simulink model "BEML_EMU_TestBench_6Car"  (R2019b)
settings: Solver=VariableStepAuto  StartTime=0.0  StopTime=inf  RelTol=1e-3
PreLoadFcn:
  | set_up_test_modelCB_6Car;
undefined symbols (not defined in the file): Common, IOControls, MaxVehicles, MotionBaseControllerInput, VehicleInputs, VehicleType, Z_CfgVehBus
libraries: TestBenchLib x583, simulink x6
(part 2 of 3)

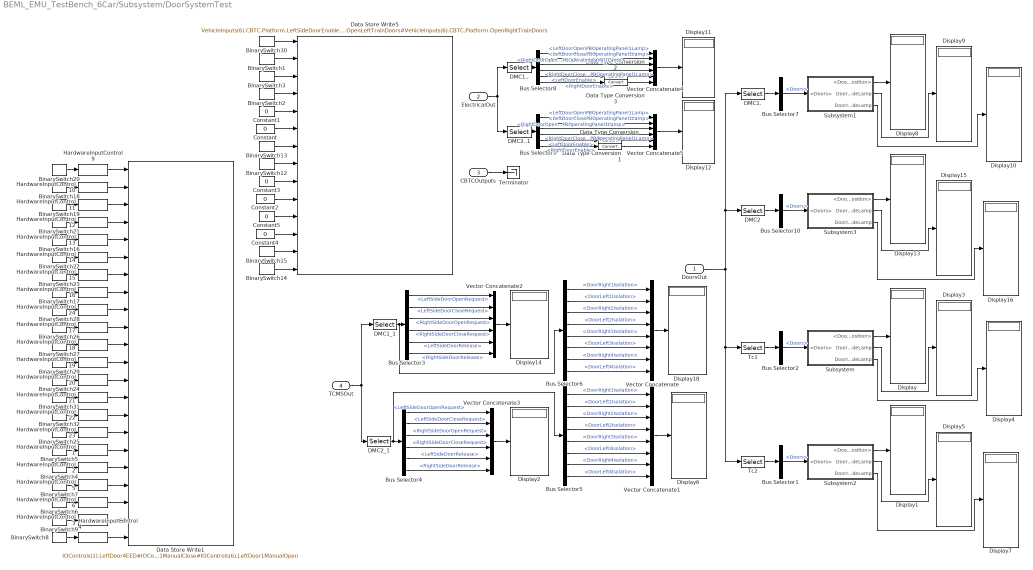
== system BEML_EMU_TestBench_6Car/Subsystem/DoorSystemTest ==
  DoorsOut : Inport
  ElectricalOut : Inport  Port=2
  CBTCOutputs : Inport  Port=3
  TCMSOut : Inport  Port=4
  BinarySwitch{1..9,12..32} (30 alike) : TestBenchLib/BinarySwitch  value=0  init_value=0  block_colour=[0 1 0]  WorkspaceVarName=0
      settings: SourceProductName=Sydac Utilities
  Bus Selector{1..2,7,10} (4 alike) : BusSelector  OutputSignals=Doors
  Bus Selector3 : BusSelector  OutputSignals=Control.DoorSystem.LeftSideDoorOpenRequest,Control.DoorSystem.LeftSideDoorCloseRequest,Control.DoorSystem.RightSideDoorOpenRequest,Control.DoorSystem.RightSideDoorCloseRequest,Control.DoorSystem.LeftSideDoorRelease,Control.DoorSystem.RightSideDoorRelease
  Bus Selector4 : BusSelector  OutputSignals=Control.DoorSystem.LeftSideDoorOpenRequest,Control.DoorSystem.LeftSideDoorCloseRequest,Control.DoorSystem.RightSideDoorOpenRequest,Control.DoorSystem.RightSideDoorCloseRequest,Control.DoorSystem.LeftSideDoorRelease,Control.DoorSystem.RightSideDoorRelease
  Bus Selector5 : BusSelector  OutputSignals=Control.DoorSystem.DoorRight1Isolation,Control.DoorSystem.DoorLeft1Isolation,Control.DoorSystem.DoorRight2Isolation,Control.DoorSystem.DoorLeft2Isolation,Control.DoorSystem.DoorRight3Isolation,Control.DoorSystem.DoorLeft3Isolation,Control.DoorSystem.DoorRight4Isolation,Control.DoorSystem.DoorLeft4Isolation
  Bus Selector6 : BusSelector  OutputSignals=Control.DoorSystem.DoorRight1Isolation,Control.DoorSystem.DoorLeft1Isolation,Control.DoorSystem.DoorRight2Isolation,Control.DoorSystem.DoorLeft2Isolation,Control.DoorSystem.DoorRight3Isolation,Control.DoorSystem.DoorLeft3Isolation,Control.DoorSystem.DoorRight4Isolation,Control.DoorSystem.DoorLeft4Isolation
  Bus Selector8 : BusSelector  OutputSignals=OutputControlStates.LeftDoorOpenPBOperatingPanel1Lamp,OutputControlStates.LeftDoorClosePBOperatingPanel1Lamp,OutputControlStates.RightDoorOpenPBOperatingPanel1Lamp,OutputControlStates.RightDoorClosePBOperatingPanel1Lamp,Doors.LeftDoorEnable,Doors.RightDoorEnable
  Bus Selector9 : BusSelector  OutputSignals=OutputControlStates.LeftDoorOpenPBOperatingPanel1Lamp,OutputControlStates.LeftDoorClosePBOperatingPanel1Lamp,OutputControlStates.RightDoorOpenPBOperatingPanel1Lamp,OutputControlStates.RightDoorClosePBOperatingPanel1Lamp,Doors.LeftDoorEnable,Doors.RightDoorEnable
  Constant{,1..5} (6 alike) : Constant  Value=0
  DMC1. : Selector  InputPortWidth=MaxVehicles  IndexOptions=Index vector (dialog)  Indices=1  OutputSizes=1
  DMC1.. : Selector  InputPortWidth=MaxVehicles  IndexOptions=Index vector (dialog)  Indices=1  OutputSizes=1
  DMC1_1 : Selector  InputPortWidth=MaxVehicles  IndexOptions=Index vector (dialog)  Indices=1  OutputSizes=1
  DMC2 : Selector  InputPortWidth=MaxVehicles  IndexOptions=Index vector (dialog)  Indices=6  OutputSizes=1
  DMC2..1 : Selector  InputPortWidth=MaxVehicles  IndexOptions=Index vector (dialog)  Indices=6  OutputSizes=1
  DMC2_1 : Selector  InputPortWidth=MaxVehicles  IndexOptions=Index vector (dialog)  Indices=6  OutputSizes=1
  Data Store Write1 : DataStoreWrite  Priority=1  DataStoreName=IOControls  DataStoreElements=IOControls(1).LeftDoor4EED#IOControls(1).LeftDoor4ManualClose#IOControls(1).LeftDoor4ManualOpen#IOControls(1).LeftDoor4Lockout#IOControls(1).RightDoor4EED#IOControls(1).RightDoor4ManualClose#IOControls(1).RightDoor4ManualOpen#IOControls(1).RightDoor4Lockout#IOControls(6).LeftDoor4EED#IOControls(6).LeftDoor4ManualClose#IOControls(6).LeftDoor4ManualOpen#IOControls(6).LeftDoor4Lockout#IOControls(6).RightDoor4EED#IOControls(6).RightDoor4ManualClose#IOControls(6).RightDoor4ManualOpen#IOControls(6).RightDoor4Lockout#IOControls(6).RightDoorEAD#IOControls(6).LeftDoorEAD#IOControls(6).RightDoor1ManualClose#IOControls(6).RightDoor1ManualOpen#IOControls(6).LeftDoor1ManualClose#IOControls(6).LeftDoor1ManualOpen
  Data Store Write5 : DataStoreWrite  Priority=1  DataStoreName=VehicleInputs  DataStoreElements=VehicleInputs(6).CBTC.Platform.LeftSideDoorEnable#VehicleInputs(6).CBTC.Platform.RightSideDoorEnable#VehicleInputs(1).CBTC.Platform.LeftSideDoorEnable#VehicleInputs(1).CBTC.Platform.RightSideDoorEnable#VehicleInputs(6).Faults.DoorCloseObstruction#VehicleInputs(6).Faults.DoorOpenObstruction#VehicleInputs(6).CBTC.OnBoard.LeftHoldDoorClose#VehicleInputs(6).CBTC.OnBoard.RightHoldDoorClose#VehicleInputs(1).Faults.DoorCloseObstruction#VehicleInputs(1).Faults.DoorOpenObstruction#VehicleInputs(2).Faults.DoorOpenObstruction#VehicleInputs(2).Faults.DoorCloseObstruction#VehicleInputs(6).CBTC.Platform.OpenLeftTrainDoors#VehicleInputs(6).CBTC.Platform.OpenRightTrainDoors
  Data Type Conversion{,1..3} (4 alike) : DataTypeConversion
  Display{,1..16,18} (18 alike) : Display
  HardwareInputControl{1..6,9..24} (22 alike) : TestBenchLib/HardwareInputControl
      settings: SourceProductName=Sydac Utilities
  Subsystem : Subsystem
  Subsystem1 : Subsystem
  Subsystem2 : Subsystem
  Subsystem3 : Subsystem
  Tc1 : Selector  InputPortWidth=MaxVehicles  IndexOptions=Index vector (dialog)  Indices=2  OutputSizes=1
  Tc2 : Selector  InputPortWidth=MaxVehicles  IndexOptions=Index vector (dialog)  Indices=5  OutputSizes=1
  Terminator : Terminator
  Vector Concatenate : Concatenate  NumInputs=8
  Vector Concatenate1 : Concatenate  NumInputs=8
  Vector Concatenate{2..5} (4 alike) : Concatenate  NumInputs=6
  wires:
  Tc1/1 -> Bus Selector2/1
  BinarySwitch30/1 -> Data Store Write5/1
  Bus Selector2/1 -> Subsystem/1(<Doors>)  "<Doors>"
  Subsystem/1(<DoorPosition>) -> Display/1
  Subsystem2/2(DoorOutsideLamp) -> Display5/1
  Bus Selector1/1 -> Subsystem2/1(<Doors>)  "<Doors>"
  Tc2/1 -> Bus Selector1/1
  DoorsOut/1 -> DMC1./1, DMC2/1, Tc1/1, Tc2/1
  BinarySwitch1/1 -> Data Store Write5/2
  DMC1_1/1 -> Bus Selector6/1, Bus Selector3/1
  TCMSOut/1 -> DMC2_1/1, DMC1_1/1
  Vector Concatenate/1 -> Display18/1
  Vector Concatenate1/1 -> Display6/1
  DMC2_1/1 -> Bus Selector5/1, Bus Selector4/1
  Bus Selector5/1 -> Vector Concatenate1/1  "<DoorRight1Isolation>"
  Bus Selector5/2 -> Vector Concatenate1/2  "<DoorLeft1Isolation>"
  Bus Selector5/3 -> Vector Concatenate1/3  "<DoorRight2Isolation>"
  Bus Selector5/4 -> Vector Concatenate1/4  "<DoorLeft2Isolation>"
  Bus Selector5/5 -> Vector Concatenate1/5  "<DoorRight3Isolation>"
  Bus Selector5/6 -> Vector Concatenate1/6  "<DoorLeft3Isolation>"
  Bus Selector5/7 -> Vector Concatenate1/7  "<DoorRight4Isolation>"
  Bus Selector5/8 -> Vector Concatenate1/8  "<DoorLeft4Isolation>"
  Bus Selector6/1 -> Vector Concatenate/1  "<DoorRight1Isolation>"
  Bus Selector6/2 -> Vector Concatenate/2  "<DoorLeft1Isolation>"
  Bus Selector6/3 -> Vector Concatenate/3  "<DoorRight2Isolation>"
  Bus Selector6/4 -> Vector Concatenate/4  "<DoorLeft2Isolation>"
  Bus Selector6/5 -> Vector Concatenate/5  "<DoorRight3Isolation>"
  Bus Selector6/6 -> Vector Concatenate/6  "<DoorLeft3Isolation>"
  Bus Selector6/7 -> Vector Concatenate/7  "<DoorRight4Isolation>"
  Bus Selector6/8 -> Vector Concatenate/8  "<DoorLeft4Isolation>"
  CBTCOutputs/1 -> Terminator/1
  Bus Selector3/1 -> Vector Concatenate2/1  "<LeftSideDoorOpenRequest>"
  Bus Selector3/2 -> Vector Concatenate2/2  "<LeftSideDoorCloseRequest>"
  Bus Selector3/3 -> Vector Concatenate2/3  "<RightSideDoorOpenRequest>"
  Bus Selector3/4 -> Vector Concatenate2/4  "<RightSideDoorCloseRequest>"
  Bus Selector3/5 -> Vector Concatenate2/5  "<LeftSideDoorRelease>"
  Bus Selector3/6 -> Vector Concatenate2/6  "<RightSideDoorRelease>"
  Vector Concatenate2/1 -> Display14/1
  Vector Concatenate3/1 -> Display2/1
  Bus Selector4/6 -> Vector Concatenate3/6  "<RightSideDoorRelease>"
  Bus Selector4/5 -> Vector Concatenate3/5  "<LeftSideDoorRelease>"
  Bus Selector4/4 -> Vector Concatenate3/4  "<RightSideDoorCloseRequest>"
  Bus Selector4/3 -> Vector Concatenate3/3  "<RightSideDoorOpenRequest>"
  Bus Selector4/2 -> Vector Concatenate3/2  "<LeftSideDoorCloseRequest>"
  Bus Selector4/1 -> Vector Concatenate3/1  "<LeftSideDoorOpenRequest>"
  ElectricalOut/1 -> DMC2..1/1, DMC1../1
  BinarySwitch2/1 -> Data Store Write5/4
  BinarySwitch3/1 -> Data Store Write5/3
  Constant1/1 -> Data Store Write5/5
  Constant/1 -> Data Store Write5/6
  BinarySwitch13/1 -> Data Store Write5/7
  BinarySwitch12/1 -> Data Store Write5/8
  Subsystem/2(DoorOutsideLamp) -> Display3/1
  Subsystem/3(DoorInsideLamp) -> Display4/1
  Subsystem2/1(<DoorPosition>) -> Display1/1
  Subsystem2/3(DoorInsideLamp) -> Display7/1
  Subsystem1/3(DoorInsideLamp) -> Display10/1
  Bus Selector7/1 -> Subsystem1/1(<Doors>)  "<Doors>"
  Subsystem1/2(DoorOutsideLamp) -> Display9/1
  Subsystem1/1(<DoorPosition>) -> Display8/1
  DMC1./1 -> Bus Selector7/1
  DMC1../1 -> Bus Selector8/1
  Bus Selector8/1 -> Vector Concatenate4/1  "<LeftDoorOpenPBOperatingPanel1Lamp>"
  Bus Selector8/2 -> Vector Concatenate4/2  "<LeftDoorClosePBOperatingPanel1Lamp>"
  Vector Concatenate4/1 -> Display11/1
  Bus Selector8/3 -> Vector Concatenate4/3  "<RightDoorOpenPBOperatingPanel1Lamp>"
  Bus Selector8/4 -> Vector Concatenate4/4  "<RightDoorClosePBOperatingPanel1Lamp>"
  Bus Selector9/4 -> Vector Concatenate5/4  "<RightDoorClosePBOperatingPanel1Lamp>"
  Bus Selector9/3 -> Vector Concatenate5/3  "<RightDoorOpenPBOperatingPanel1Lamp>"
  Vector Concatenate5/1 -> Display12/1
  Bus Selector9/2 -> Vector Concatenate5/2  "<LeftDoorClosePBOperatingPanel1Lamp>"
  Bus Selector9/1 -> Vector Concatenate5/1  "<LeftDoorOpenPBOperatingPanel1Lamp>"
  DMC2..1/1 -> Bus Selector9/1
  Constant2/1 -> Data Store Write5/10
  Constant3/1 -> Data Store Write5/9
  Constant5/1 -> Data Store Write5/11
  Constant4/1 -> Data Store Write5/12
  BinarySwitch14/1 -> Data Store Write5/14
  BinarySwitch15/1 -> Data Store Write5/13
  DMC2/1 -> Bus Selector10/1
  Subsystem3/1(<DoorPosition>) -> Display13/1
  Subsystem3/3(DoorInsideLamp) -> Display16/1
  Subsystem3/2(DoorOutsideLamp) -> Display15/1
  Bus Selector10/1 -> Subsystem3/1(<Doors>)  "<Doors>"
  Bus Selector8/5 -> Data Type Conversion2/1  "<LeftDoorEnable>"
  Bus Selector8/6 -> Data Type Conversion3/1  "<RightDoorEnable>"
  Bus Selector9/5 -> Data Type Conversion/1  "<LeftDoorEnable>"
  Bus Selector9/6 -> Data Type Conversion1/1  "<RightDoorEnable>"
  Data Type Conversion/1 -> Vector Concatenate5/5
  Data Type Conversion1/1 -> Vector Concatenate5/6
  Data Type Conversion2/1 -> Vector Concatenate4/5
  Data Type Conversion3/1 -> Vector Concatenate4/6
  BinarySwitch23/1 -> HardwareInputControl15/1
  BinarySwitch22/1 -> HardwareInputControl14/1
  BinarySwitch16/1 -> HardwareInputControl13/1
  HardwareInputControl13/1 -> Data Store Write1/5
  HardwareInputControl14/1 -> Data Store Write1/6
  HardwareInputControl15/1 -> Data Store Write1/7
  BinarySwitch17/1 -> HardwareInputControl16/1
  HardwareInputControl16/1 -> Data Store Write1/8
  HardwareInputControl12/1 -> Data Store Write1/4
  BinarySwitch21/1 -> HardwareInputControl12/1
  HardwareInputControl11/1 -> Data Store Write1/3
  HardwareInputControl10/1 -> Data Store Write1/2
  HardwareInputControl9/1 -> Data Store Write1/1
  BinarySwitch20/1 -> HardwareInputControl9/1
  BinarySwitch18/1 -> HardwareInputControl10/1
  BinarySwitch19/1 -> HardwareInputControl11/1
  BinarySwitch27/1 -> HardwareInputControl18/1
  BinarySwitch26/1 -> HardwareInputControl17/1
  BinarySwitch28/1 -> HardwareInputControl24/1
  HardwareInputControl24/1 -> Data Store Write1/9
  HardwareInputControl17/1 -> Data Store Write1/10
  HardwareInputControl18/1 -> Data Store Write1/11
  BinarySwitch29/1 -> HardwareInputControl19/1
  HardwareInputControl19/1 -> Data Store Write1/12
  HardwareInputControl23/1 -> Data Store Write1/16
  BinarySwitch25/1 -> HardwareInputControl23/1
  HardwareInputControl22/1 -> Data Store Write1/15
  HardwareInputControl21/1 -> Data Store Write1/14
  HardwareInputControl20/1 -> Data Store Write1/13
  BinarySwitch24/1 -> HardwareInputControl20/1
  BinarySwitch31/1 -> HardwareInputControl21/1
  BinarySwitch32/1 -> HardwareInputControl22/1
  BinarySwitch5/1 -> HardwareInputControl1/1
  HardwareInputControl1/1 -> Data Store Write1/17
  BinarySwitch4/1 -> HardwareInputControl2/1
  HardwareInputControl2/1 -> Data Store Write1/18
  HardwareInputControl4/1 -> Data Store Write1/22
  BinarySwitch8/1 -> HardwareInputControl4/1
  HardwareInputControl3/1 -> Data Store Write1/21
  BinarySwitch9/1 -> HardwareInputControl3/1
  BinarySwitch7/1 -> HardwareInputControl5/1
  HardwareInputControl5/1 -> Data Store Write1/19
  BinarySwitch6/1 -> HardwareInputControl6/1
  HardwareInputControl6/1 -> Data Store Write1/20

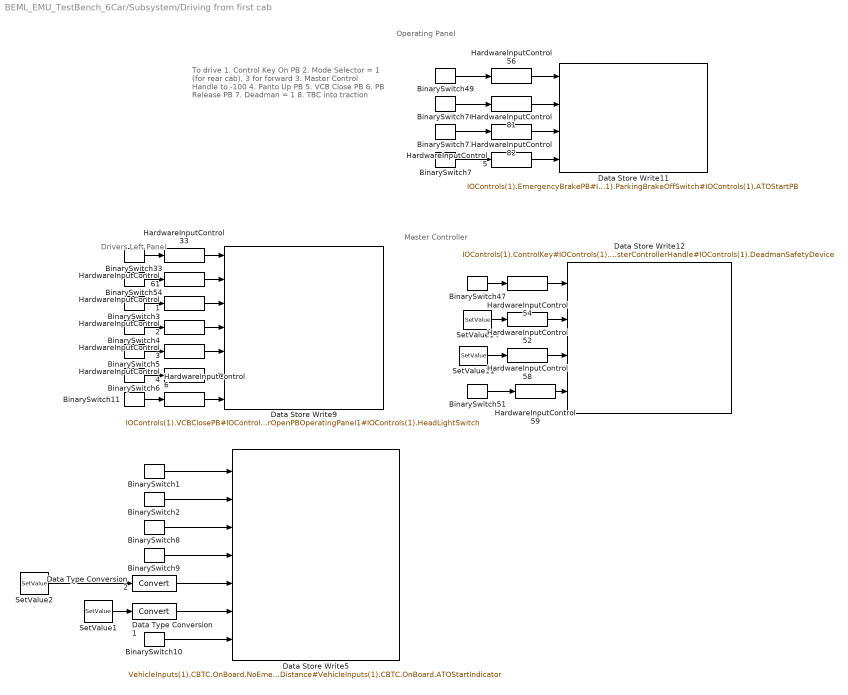
== system BEML_EMU_TestBench_6Car/Subsystem/Driving from first cab ==
  note: Master Controller
  note: Drivers Left Panel
  note: To drive
      | 1. Control Key On PB
      | 2. Mode Selector = 1 (for rear cab), 3 for forward
      | 3. Master Control Handle to -100
      | 4. Panto Up PB
      | 5. VCB Close PB
      | 6. PB Release PB
      | 7. Deadman = 1
      | 8. TBC into traction
  note: Operating Panel
  BinarySwitch{1..2,8,51} (4 alike) : TestBenchLib/BinarySwitch  value=1  init_value=1  block_colour=[0 1 0]  WorkspaceVarName=0
      settings: SourceProductName=Sydac Utilities
  BinarySwitch{3..7,9..11,33,47,49,54,70..71} (14 alike) : TestBenchLib/BinarySwitch  value=0  init_value=0  block_colour=[0 1 0]  WorkspaceVarName=0
      settings: SourceProductName=Sydac Utilities
  Data Store Write11 : DataStoreWrite  Priority=1  DataStoreName=IOControls  DataStoreElements=IOControls(1).EmergencyBrakePB#IOControls(1).ParkingBrakeOnSwitch#IOControls(1).ParkingBrakeOffSwitch#IOControls(1).ATOStartPB
  Data Store Write12 : DataStoreWrite  Priority=1  DataStoreName=IOControls  DataStoreElements=IOControls(1).ControlKey#IOControls(1).ModeSelector#IOControls(1).MasterControllerHandle#IOControls(1).DeadmanSafetyDevice
  Data Store Write5 : DataStoreWrite  Priority=1  DataStoreName=VehicleInputs  DataStoreElements=VehicleInputs(1).CBTC.OnBoard.NoEmergencyBrakeOrder#VehicleInputs(1).CBTC.OnBoard.NoServiceBrakeOrder#VehicleInputs(1).CBTC.OnBoard.ImmobilisationState#VehicleInputs(1).CBTC.OnBoard.ATOState#VehicleInputs(1).CBTC.OnBoard.ATOPermittedSpeed#VehicleInputs(1).CBTC.OnBoard.ATOPermittedDistance#VehicleInputs(1).CBTC.OnBoard.ATOStartIndicator
  Data Store Write9 : DataStoreWrite  Priority=1  DataStoreName=IOControls  DataStoreElements=IOControls(1).VCBClosePB#IOControls(1).PantoUpPB#IOControls(1).LeftDoorClosePBOperatingPanel1#IOControls(1).RightDoorClosePBOperatingPanel1#IOControls(1).LeftDoorOpenPBOperatingPanel1#IOControls(1).RightDoorOpenPBOperatingPanel1#IOControls(1).HeadLightSwitch
  Data Type Conversion1 : DataTypeConversion
  Data Type Conversion2 : DataTypeConversion
  HardwareInputControl{1..6,33,52,54,56,58..59,61,81..82} (15 alike) : TestBenchLib/HardwareInputControl
      settings: SourceProductName=Sydac Utilities
  SetValue1 : TestBenchLib/SetValue  value=500  init_value=500  WorkspaceVarName=0
      settings: SourceProductName=Sydac Utilities
  SetValue11 : TestBenchLib/SetValue  value=-100  init_value=-100  WorkspaceVarName=0
      settings: SourceProductName=Sydac Utilities
  SetValue14 : TestBenchLib/SetValue  value=0  init_value=0  WorkspaceVarName=0
      settings: SourceProductName=Sydac Utilities
  SetValue2 : TestBenchLib/SetValue  value=0  init_value=0  WorkspaceVarName=0
      settings: SourceProductName=Sydac Utilities
  wires:
  HardwareInputControl81/1 -> Data Store Write11/2
  HardwareInputControl56/1 -> Data Store Write11/1
  HardwareInputControl58/1 -> Data Store Write12/3
  BinarySwitch54/1 -> HardwareInputControl61/1
  HardwareInputControl61/1 -> Data Store Write9/2
  HardwareInputControl33/1 -> Data Store Write9/1
  SetValue11/1 -> HardwareInputControl58/1
  HardwareInputControl54/1 -> Data Store Write12/1
  HardwareInputControl82/1 -> Data Store Write11/3
  BinarySwitch47/1 -> HardwareInputControl54/1
  HardwareInputControl59/1 -> Data Store Write12/4
  BinarySwitch51/1 -> HardwareInputControl59/1
  BinarySwitch33/1 -> HardwareInputControl33/1
  SetValue14/1 -> HardwareInputControl52/1
  BinarySwitch49/1 -> HardwareInputControl56/1
  BinarySwitch71/1 -> HardwareInputControl82/1
  BinarySwitch70/1 -> HardwareInputControl81/1
  HardwareInputControl52/1 -> Data Store Write12/2
  BinarySwitch1/1 -> Data Store Write5/1
  BinarySwitch2/1 -> Data Store Write5/2
  BinarySwitch3/1 -> HardwareInputControl1/1
  HardwareInputControl1/1 -> Data Store Write9/3
  HardwareInputControl2/1 -> Data Store Write9/4
  BinarySwitch4/1 -> HardwareInputControl2/1
  BinarySwitch6/1 -> HardwareInputControl4/1
  HardwareInputControl4/1 -> Data Store Write9/6
  HardwareInputControl3/1 -> Data Store Write9/5
  BinarySwitch5/1 -> HardwareInputControl3/1
  BinarySwitch7/1 -> HardwareInputControl5/1
  HardwareInputControl5/1 -> Data Store Write11/4
  BinarySwitch8/1 -> Data Store Write5/3
  BinarySwitch9/1 -> Data Store Write5/4
  BinarySwitch10/1 -> Data Store Write5/7
  SetValue2/1 -> Data Type Conversion2/1
  Data Type Conversion2/1 -> Data Store Write5/5
  SetValue1/1 -> Data Type Conversion1/1
  Data Type Conversion1/1 -> Data Store Write5/6
  HardwareInputControl6/1 -> Data Store Write9/7
  BinarySwitch11/1 -> HardwareInputControl6/1

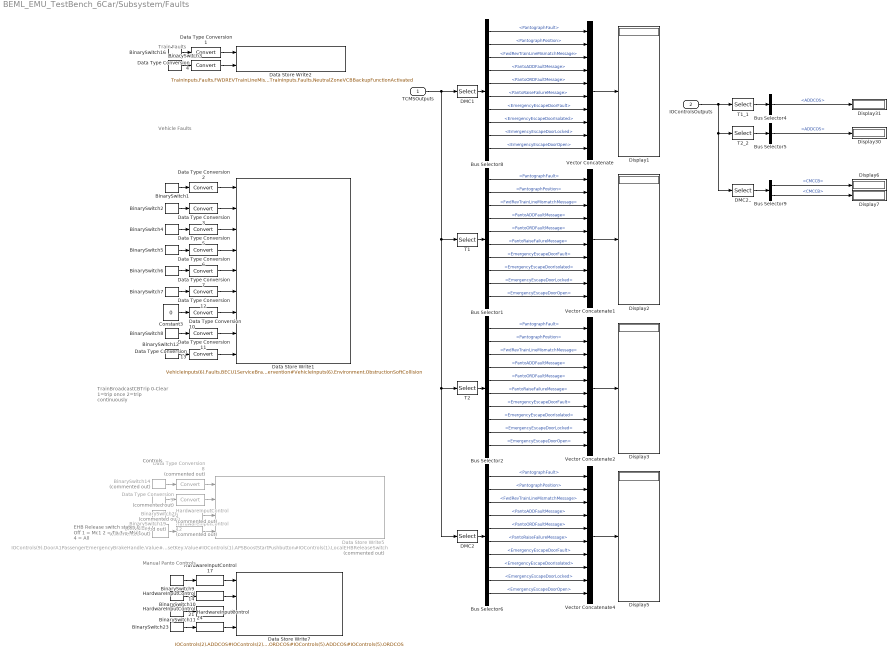
== system BEML_EMU_TestBench_6Car/Subsystem/Faults ==
  note: TrainBroadcastCBTrip
      | 0-Clear
      | 1=trip once
      | 2=trip continuously
  note: EHB Release switch states
      | 0 = Off
      | 1 = Mc1
      | 2 = Tp
      | 3 = Msc1
      | 4 = All
  note: Vehicle Faults
  note: Train Faults
  note: Controls
  note: Manual Panto Controls
  TCMSOutputs : Inport
  IOControlsOutputs : Inport  Port=2
  BinarySwitch{1..12,16,23} (14 alike) : TestBenchLib/BinarySwitch  value=0  init_value=0  block_colour=[0 1 0]  WorkspaceVarName=0
      settings: SourceProductName=Sydac Utilities
  BinarySwitch14 : TestBenchLib/BinarySwitch  Commented=on  value=0  init_value=0  block_colour=[0 1 0]  WorkspaceVarName=0
      settings: SourceProductName=Sydac Utilities
  BinarySwitch19 : TestBenchLib/BinarySwitch  Commented=on  value=0  init_value=0  block_colour=[0 1 0]  WorkspaceVarName=0
      settings: SourceProductName=Sydac Utilities
  BinarySwitch20 : TestBenchLib/BinarySwitch  Commented=on  value=0  init_value=0  block_colour=[0 1 0]  WorkspaceVarName=0
      settings: SourceProductName=Sydac Utilities
  Bus Selector{1..2,6,8} (4 alike) : BusSelector  OutputSignals=Display.PantographSystem.PantographFault,Display.PantographSystem.PantographPosition,Control.ElectricalSystem.FwdRevTrainLineMismatchMessage,Display.PantographSystem.PantoADDFaultMessage,Display.PantographSystem.PantoORDFaultMessage,Display.PantographSystem.PantoRaiseFailureMessage,Display.DoorSystem.EmergencyEscapeDoorFault,Display.DoorSystem.EmergencyEscapeDoorIsolated,Display.DoorSystem.EmergencyEscapeDoorLocked,Display.DoorSystem.EmergencyEscapeDoorOpen
  Bus Selector4 : BusSelector  OutputSignals=InputStates.ADDCOS
  Bus Selector5 : BusSelector  OutputSignals=InputStates.ADDCOS
  Bus Selector9 : BusSelector  OutputSignals=InputStates.CMCCB,MCBTripStates.CMCCB
  Constant3 : Constant  Value=0
  DMC1 : Selector  InputPortWidth=MaxVehicles  IndexOptions=Index vector (dialog)  Indices=1  OutputSizes=1
  DMC2 : Selector  InputPortWidth=MaxVehicles  IndexOptions=Index vector (dialog)  Indices=6  OutputSizes=1
  DMC2.. : Selector  InputPortWidth=MaxVehicles  IndexOptions=Index vector (dialog)  Indices=6  OutputSizes=1
  Data Store Write1 : DataStoreWrite  Priority=1  DataStoreName=VehicleInputs  DataStoreElements=VehicleInputs(6).Faults.BECU1ServiceBrakeFailure#VehicleInputs(6).Faults.BECU1FailureAllSpeedSensors#VehicleInputs(6).Faults.BECU1BrakeNotApplied#VehicleInputs(5).Faults.BECULowRPressure#VehicleInputs(6).Faults.BECULowRPressure#VehicleInputs(6).Faults.BECU1AxleLockedWheelSet1#VehicleInputs(6).Faults.ODDFailure#VehicleInputs(5).Faults.PantographDownForORDIntervention#VehicleInputs(6).Environment.ObstructionSoftCollision
  Data Store Write2 : DataStoreWrite  Priority=1  DataStoreName=TrainInputs  DataStoreElements=TrainInputs.Faults.FWDREVTrainLineMismatch#TrainInputs.Faults.NeutralZoneVCBBackupFunctionActivated
  Data Store Write5 : DataStoreWrite  Priority=1  Commented=on  DataStoreName=IOControls  DataStoreElements=IOControls(9).DoorA1PassengerEmergencyBrakeHandle.Value#IOControls(9).DoorA1PassengerEmergencyBrakeHandleResetKey.Value#IOControls(1).APSBoostStartPushbutton#IOControls(1).LocalEHBReleaseSwitch
  Data Store Write7 : DataStoreWrite  Priority=1  DataStoreName=IOControls  DataStoreElements=IOControls(2).ADDCOS#IOControls(2).ORDCOS#IOControls(5).ADDCOS#IOControls(5).ORDCOS
  Data Type Conversion{1..7,10..13} (11 alike) : DataTypeConversion
  Data Type Conversion8 : DataTypeConversion  Commented=on
  Data Type Conversion9 : DataTypeConversion  Commented=on
  Display{1..3,5..7,30..31} (8 alike) : Display
  HardwareInputControl1 : TestBenchLib/HardwareInputControl  Commented=on
      settings: SourceProductName=Sydac Utilities
  HardwareInputControl12 : TestBenchLib/HardwareInputControl  Commented=on
      settings: SourceProductName=Sydac Utilities
  HardwareInputControl{14,17,21,24} (4 alike) : TestBenchLib/HardwareInputControl
      settings: SourceProductName=Sydac Utilities
  SetValue4 : TestBenchLib/SetValue  Commented=on  value=0  init_value=0  WorkspaceVarName=0
      settings: SourceProductName=Sydac Utilities
  T1 : Selector  InputPortWidth=MaxVehicles  IndexOptions=Index vector (dialog)  Indices=2  OutputSizes=1
  T1_1 : Selector  InputPortWidth=MaxVehicles  IndexOptions=Index vector (dialog)  Indices=2  OutputSizes=1
  T2 : Selector  InputPortWidth=MaxVehicles  IndexOptions=Index vector (dialog)  Indices=5  OutputSizes=1
  T2_2 : Selector  InputPortWidth=MaxVehicles  IndexOptions=Index vector (dialog)  Indices=5  OutputSizes=1
  Vector Concatenate{,1..2,4} (4 alike) : Concatenate  NumInputs=10
  wires:
  Data Type Conversion1/1 -> Data Store Write2/1
  BinarySwitch16/1 -> Data Type Conversion1/1
  DMC1/1 -> Bus Selector8/1
  IOControlsOutputs/1 -> DMC2../1, T2_2/1, T1_1/1
  T1_1/1 -> Bus Selector4/1
  T2_2/1 -> Bus Selector5/1
  Bus Selector5/1 -> Display30/1  "<ADDCOS>"
  Bus Selector4/1 -> Display31/1  "<ADDCOS>"
  BinarySwitch14/1 -> Data Type Conversion8/1
  Data Type Conversion9/1 -> Data Store Write5/2
  Data Type Conversion8/1 -> Data Store Write5/1
  BinarySwitch20/1 -> Data Type Conversion9/1
  HardwareInputControl12/1 -> Data Store Write5/3
  BinarySwitch19/1 -> HardwareInputControl12/1
  SetValue4/1 -> HardwareInputControl1/1
  HardwareInputControl1/1 -> Data Store Write5/4
  TCMSOutputs/1 -> DMC2/1, T2/1, T1/1, DMC1/1
  HardwareInputControl17/1 -> Data Store Write7/1
  HardwareInputControl14/1 -> Data Store Write7/2
  BinarySwitch23/1 -> HardwareInputControl24/1
  BinarySwitch11/1 -> HardwareInputControl21/1
  BinarySwitch9/1 -> HardwareInputControl17/1
  HardwareInputControl21/1 -> Data Store Write7/3
  BinarySwitch10/1 -> HardwareInputControl14/1
  HardwareInputControl24/1 -> Data Store Write7/4
  Bus Selector8/1 -> Vector Concatenate/1  "<PantographFault>"
  Bus Selector8/2 -> Vector Concatenate/2  "<PantographPosition>"
  Bus Selector8/3 -> Vector Concatenate/3  "<FwdRevTrainLineMismatchMessage>"
  Bus Selector8/4 -> Vector Concatenate/4  "<PantoADDFaultMessage>"
  Bus Selector8/5 -> Vector Concatenate/5  "<PantoORDFaultMessage>"
  Bus Selector8/6 -> Vector Concatenate/6  "<PantoRaiseFailureMessage>"
  Bus Selector8/7 -> Vector Concatenate/7  "<EmergencyEscapeDoorFault>"
  Bus Selector8/8 -> Vector Concatenate/8  "<EmergencyEscapeDoorIsolated>"
  Bus Selector8/9 -> Vector Concatenate/9  "<EmergencyEscapeDoorLocked>"
  Bus Selector8/10 -> Vector Concatenate/10  "<EmergencyEscapeDoorOpen>"
  Vector Concatenate/1 -> Display1/1
  Vector Concatenate1/1 -> Display2/1
  Bus Selector1/10 -> Vector Concatenate1/10  "<EmergencyEscapeDoorOpen>"
  Bus Selector1/9 -> Vector Concatenate1/9  "<EmergencyEscapeDoorLocked>"
  Bus Selector1/8 -> Vector Concatenate1/8  "<EmergencyEscapeDoorIsolated>"
  Bus Selector1/7 -> Vector Concatenate1/7  "<EmergencyEscapeDoorFault>"
  Bus Selector1/6 -> Vector Concatenate1/6  "<PantoRaiseFailureMessage>"
  Bus Selector1/5 -> Vector Concatenate1/5  "<PantoORDFaultMessage>"
  Bus Selector1/4 -> Vector Concatenate1/4  "<PantoADDFaultMessage>"
  Bus Selector1/3 -> Vector Concatenate1/3  "<FwdRevTrainLineMismatchMessage>"
  Bus Selector1/2 -> Vector Concatenate1/2  "<PantographPosition>"
  Bus Selector1/1 -> Vector Concatenate1/1  "<PantographFault>"
  T1/1 -> Bus Selector1/1
  T2/1 -> Bus Selector2/1
  Bus Selector2/1 -> Vector Concatenate2/1  "<PantographFault>"
  Bus Selector2/2 -> Vector Concatenate2/2  "<PantographPosition>"
  Bus Selector2/3 -> Vector Concatenate2/3  "<FwdRevTrainLineMismatchMessage>"
  Bus Selector2/4 -> Vector Concatenate2/4  "<PantoADDFaultMessage>"
  Bus Selector2/5 -> Vector Concatenate2/5  "<PantoORDFaultMessage>"
  Bus Selector2/6 -> Vector Concatenate2/6  "<PantoRaiseFailureMessage>"
  Bus Selector2/7 -> Vector Concatenate2/7  "<EmergencyEscapeDoorFault>"
  Bus Selector2/8 -> Vector Concatenate2/8  "<EmergencyEscapeDoorIsolated>"
  Bus Selector2/9 -> Vector Concatenate2/9  "<EmergencyEscapeDoorLocked>"
  Bus Selector2/10 -> Vector Concatenate2/10  "<EmergencyEscapeDoorOpen>"
  Vector Concatenate2/1 -> Display3/1
  DMC2/1 -> Bus Selector6/1
  Bus Selector6/1 -> Vector Concatenate4/1  "<PantographFault>"
  Bus Selector6/2 -> Vector Concatenate4/2  "<PantographPosition>"
  Bus Selector6/3 -> Vector Concatenate4/3  "<FwdRevTrainLineMismatchMessage>"
  Bus Selector6/4 -> Vector Concatenate4/4  "<PantoADDFaultMessage>"
  Bus Selector6/5 -> Vector Concatenate4/5  "<PantoORDFaultMessage>"
  Bus Selector6/6 -> Vector Concatenate4/6  "<PantoRaiseFailureMessage>"
  Bus Selector6/7 -> Vector Concatenate4/7  "<EmergencyEscapeDoorFault>"
  Bus Selector6/8 -> Vector Concatenate4/8  "<EmergencyEscapeDoorIsolated>"
  Bus Selector6/9 -> Vector Concatenate4/9  "<EmergencyEscapeDoorLocked>"
  Bus Selector6/10 -> Vector Concatenate4/10  "<EmergencyEscapeDoorOpen>"
  Vector Concatenate4/1 -> Display5/1
  DMC2../1 -> Bus Selector9/1
  Bus Selector9/1 -> Display6/1  "<CMCCB>"
  Bus Selector9/2 -> Display7/1  "<CMCCB>"
  BinarySwitch3/1 -> Data Type Conversion4/1
  Data Type Conversion4/1 -> Data Store Write2/2
  BinarySwitch1/1 -> Data Type Conversion2/1
  Data Type Conversion2/1 -> Data Store Write1/1
  Data Type Conversion3/1 -> Data Store Write1/2
  BinarySwitch2/1 -> Data Type Conversion3/1
  BinarySwitch4/1 -> Data Type Conversion5/1
  Data Type Conversion5/1 -> Data Store Write1/3
  Data Type Conversion6/1 -> Data Store Write1/4
  BinarySwitch5/1 -> Data Type Conversion6/1
  Data Type Conversion10/1 -> Data Store Write1/7
  Constant3/1 -> Data Type Conversion10/1
  BinarySwitch6/1 -> Data Type Conversion7/1
  Data Type Conversion7/1 -> Data Store Write1/5
  Data Type Conversion12/1 -> Data Store Write1/6
  BinarySwitch7/1 -> Data Type Conversion12/1
  BinarySwitch8/1 -> Data Type Conversion11/1
  Data Type Conversion11/1 -> Data Store Write1/8
  Data Type Conversion13/1 -> Data Store Write1/9
  BinarySwitch12/1 -> Data Type Conversion13/1

== system BEML_EMU_TestBench_6Car/Subsystem/For Each Subsystem ==
  In1 : Inport  Partition=on  PartitionDimension=1  PartitionWidth=1  PartitionOffset=0
  Bus Selector : BusSelector  OutputSignals=Inertia.BogieSupportedMass
  For Each : ForEach  DisableCoverage=on
  Out1 : Outport  ConcatenationDimension=1
  wires:
  In1/1 -> Bus Selector/1
  Bus Selector/1 -> Out1/1  "<BogieSupportedMass>"

== system BEML_EMU_TestBench_6Car/Subsystem/IOControlsInput ==
  note: RampCover opens emergency door
  BinarySwitch{1..6,53} (7 alike) : TestBenchLib/BinarySwitch  value=0  init_value=0  block_colour=[0 1 0]  WorkspaceVarName=0
      settings: SourceProductName=Sydac Utilities
  BinarySwitch7 : TestBenchLib/BinarySwitch  value=1  init_value=1  block_colour=[0 1 0]  WorkspaceVarName=0
      settings: SourceProductName=Sydac Utilities
  BinarySwitch8 : TestBenchLib/BinarySwitch  value=1  init_value=1  block_colour=[0 1 0]  WorkspaceVarName=0
      settings: SourceProductName=Sydac Utilities
  BinarySwitch9 : TestBenchLib/BinarySwitch  value=1  init_value=1  block_colour=[0 1 0]  WorkspaceVarName=0
      settings: SourceProductName=Sydac Utilities
  Data Store Write1 : DataStoreWrite  Priority=1  DataStoreName=IOControls  DataStoreElements=IOControls(6).ParkingBrakeManualReleaseBogie1Handle1#IOControls(6).ParkingBrakeManualReleaseBogie1Handle2#IOControls(6).ParkingBrakeManualReleaseBogie2Handle1#IOControls(6).ParkingBrakeManualReleaseBogie2Handle2#IOControls(6).DriversBackDoor#IOControls(1).DriversBackDoor#IOControls(6).SafetyCover#IOControls(6).DummyCover#IOControls(6).RampCoverLockingLever
  Data Store Write10 : DataStoreWrite  Priority=1  DataStoreName=IOControls  DataStoreElements=IOControls(6).RampCover
  HardwareInputControl{1..9,33} (10 alike) : TestBenchLib/HardwareInputControl
      settings: SourceProductName=Sydac Utilities
  wires:
  BinarySwitch53/1 -> HardwareInputControl33/1
  HardwareInputControl33/1 -> Data Store Write10/1
  HardwareInputControl1/1 -> Data Store Write1/1
  BinarySwitch1/1 -> HardwareInputControl1/1
  BinarySwitch2/1 -> HardwareInputControl2/1
  HardwareInputControl2/1 -> Data Store Write1/2
  HardwareInputControl4/1 -> Data Store Write1/4
  BinarySwitch4/1 -> HardwareInputControl4/1
  BinarySwitch3/1 -> HardwareInputControl3/1
  HardwareInputControl3/1 -> Data Store Write1/3
  HardwareInputControl5/1 -> Data Store Write1/5
  BinarySwitch5/1 -> HardwareInputControl5/1
  BinarySwitch6/1 -> HardwareInputControl6/1
  HardwareInputControl6/1 -> Data Store Write1/6
  HardwareInputControl9/1 -> Data Store Write1/9
  BinarySwitch9/1 -> HardwareInputControl9/1
  BinarySwitch8/1 -> HardwareInputControl8/1
  HardwareInputControl8/1 -> Data Store Write1/8
  BinarySwitch7/1 -> HardwareInputControl7/1
  HardwareInputControl7/1 -> Data Store Write1/7

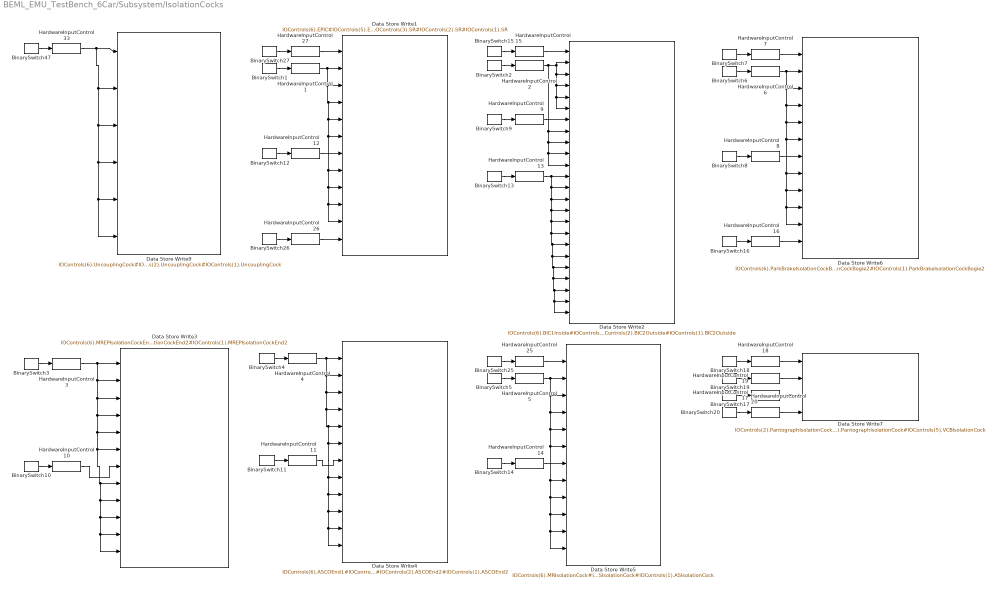
== system BEML_EMU_TestBench_6Car/Subsystem/IsolationCocks ==
  BinarySwitch{1..20,25..27,47} (24 alike) : TestBenchLib/BinarySwitch  value=1  init_value=1  block_colour=[0 1 0]  WorkspaceVarName=0
      settings: SourceProductName=Sydac Utilities
  Data Store Write1 : DataStoreWrite  Priority=1  DataStoreName=IOControls  DataStoreElements=IOControls(6).EPIC#IOControls(5).EPIC#IOControls(4).EPIC#IOControls(3).EPIC#IOControls(2).EPIC#IOControls(1).EPIC#IOControls(6).SR#IOControls(5).SR#IOControls(4).SR#IOControls(3).SR#IOControls(2).SR#IOControls(1).SR
  Data Store Write2 : DataStoreWrite  Priority=1  DataStoreName=IOControls  DataStoreElements=IOControls(6).BIC1Inside#IOControls(5).BIC1Inside#IOControls(4).BIC1Inside#IOControls(3).BIC1Inside#IOControls(2).BIC1Inside#IOControls(1).BIC1Inside#IOControls(6).BIC1Outside#IOControls(5).BIC1Outside#IOControls(4).BIC1Outside#IOControls(3).BIC1Outside#IOControls(2).BIC1Outside#IOControls(1).BIC1Outside#IOControls(6).BIC2Inside#IOControls(5).BIC2Inside#IOControls(4).BIC2Inside#IOControls(3).BIC2Inside#IOControls(2).BIC2Inside#IOControls(1).BIC2Inside#IOControls(6).BIC2Outside#IOControls(5).BIC2Outside#IOControls(4).BIC2Outside#IOControls(3).BIC2Outside#IOControls(2).BIC2Outside#IOControls(1).BIC2Outside
  Data Store Write3 : DataStoreWrite  Priority=1  DataStoreName=IOControls  DataStoreElements=IOControls(6).MREPIsolationCockEnd1#IOControls(5).MREPIsolationCockEnd1#IOControls(4).MREPIsolationCockEnd1#IOControls(3).MREPIsolationCockEnd1#IOControls(2).MREPIsolationCockEnd1#IOControls(1).MREPIsolationCockEnd1#IOControls(6).MREPIsolationCockEnd2#IOControls(5).MREPIsolationCockEnd2#IOControls(4).MREPIsolationCockEnd2#IOControls(3).MREPIsolationCockEnd2#IOControls(2).MREPIsolationCockEnd2#IOControls(1).MREPIsolationCockEnd2
  Data Store Write4 : DataStoreWrite  Priority=1  DataStoreName=IOControls  DataStoreElements=IOControls(6).ASCOEnd1#IOControls(5).ASCOEnd1#IOControls(4).ASCOEnd1#IOControls(3).ASCOEnd1#IOControls(2).ASCOEnd1#IOControls(1).ASCOEnd1#IOControls(6).ASCOEnd2#IOControls(5).ASCOEnd2#IOControls(4).ASCOEnd2#IOControls(3).ASCOEnd2#IOControls(2).ASCOEnd2#IOControls(1).ASCOEnd2
  Data Store Write5 : DataStoreWrite  Priority=1  DataStoreName=IOControls  DataStoreElements=IOControls(6).MRIsolationCock#IOControls(5).MRIsolationCock#IOControls(4).MRIsolationCock#IOControls(3).MRIsolationCock#IOControls(2).MRIsolationCock#IOControls(1).MRIsolationCock#IOControls(6).ASIsolationCock#IOControls(5).ASIsolationCock#IOControls(4).ASIsolationCock#IOControls(3).ASIsolationCock#IOControls(2).ASIsolationCock#IOControls(1).ASIsolationCock
  Data Store Write6 : DataStoreWrite  Priority=1  DataStoreName=IOControls  DataStoreElements=IOControls(6).ParkBrakeIsolationCockBogie1#IOControls(5).ParkBrakeIsolationCockBogie1#IOControls(4).ParkBrakeIsolationCockBogie1#IOControls(3).ParkBrakeIsolationCockBogie1#IOControls(2).ParkBrakeIsolationCockBogie1#IOControls(1).ParkBrakeIsolationCockBogie1#IOControls(6).ParkBrakeIsolationCockBogie2#IOControls(5).ParkBrakeIsolationCockBogie2#IOControls(4).ParkBrakeIsolationCockBogie2#IOControls(3).ParkBrakeIsolationCockBogie2#IOControls(2).ParkBrakeIsolationCockBogie2#IOControls(1).ParkBrakeIsolationCockBogie2
  Data Store Write7 : DataStoreWrite  Priority=1  DataStoreName=IOControls  DataStoreElements=IOControls(2).PantographIsolationCock#IOControls(2).VCBIsolationCock#IOControls(5).PantographIsolationCock#IOControls(5).VCBIsolationCock
  Data Store Write9 : DataStoreWrite  Priority=1  DataStoreName=IOControls  DataStoreElements=IOControls(6).UncouplingCock#IOControls(5).UncouplingCock#IOControls(4).UncouplingCock#IOControls(3).UncouplingCock#IOControls(2).UncouplingCock#IOControls(1).UncouplingCock
  HardwareInputControl{1..20,25..27,33} (24 alike) : TestBenchLib/HardwareInputControl
      settings: SourceProductName=Sydac Utilities
  wires:
  BinarySwitch47/1 -> HardwareInputControl33/1
  HardwareInputControl33/1 -> Data Store Write9/6, Data Store Write9/5, Data Store Write9/4, Data Store Write9/3, Data Store Write9/2, Data Store Write9/1
  BinarySwitch1/1 -> HardwareInputControl1/1
  HardwareInputControl1/1 -> Data Store Write1/8, Data Store Write1/9, Data Store Write1/10, Data Store Write1/11, Data Store Write1/6, Data Store Write1/5, Data Store Write1/4, Data Store Write1/3, Data Store Write1/2
  BinarySwitch3/1 -> HardwareInputControl3/1
  HardwareInputControl3/1 -> Data Store Write3/2, Data Store Write3/3, Data Store Write3/5, Data Store Write3/6, Data Store Write3/9, Data Store Write3/12, Data Store Write3/11, Data Store Write3/10, Data Store Write3/8, Data Store Write3/4, Data Store Write3/1
  BinarySwitch4/1 -> HardwareInputControl4/1
  HardwareInputControl4/1 -> Data Store Write4/9, Data Store Write4/12, Data Store Write4/11, Data Store Write4/10, Data Store Write4/8, Data Store Write4/6, Data Store Write4/5, Data Store Write4/4, Data Store Write4/3, Data Store Write4/2, Data Store Write4/1
  BinarySwitch5/1 -> HardwareInputControl5/1
  HardwareInputControl6/1 -> Data Store Write6/2, Data Store Write6/3, Data Store Write6/4, Data Store Write6/5, Data Store Write6/6, Data Store Write6/8, Data Store Write6/9, Data Store Write6/10, Data Store Write6/11
  BinarySwitch6/1 -> HardwareInputControl6/1
  HardwareInputControl5/1 -> Data Store Write5/2, Data Store Write5/3, Data Store Write5/4, Data Store Write5/5, Data Store Write5/6, Data Store Write5/8, Data Store Write5/9, Data Store Write5/10, Data Store Write5/11, Data Store Write5/12
  BinarySwitch7/1 -> HardwareInputControl7/1
  HardwareInputControl7/1 -> Data Store Write6/1
  HardwareInputControl8/1 -> Data Store Write6/7
  BinarySwitch8/1 -> HardwareInputControl8/1
  BinarySwitch10/1 -> HardwareInputControl10/1
  HardwareInputControl10/1 -> Data Store Write3/7
  BinarySwitch11/1 -> HardwareInputControl11/1
  HardwareInputControl11/1 -> Data Store Write4/7
  BinarySwitch12/1 -> HardwareInputControl12/1
  HardwareInputControl12/1 -> Data Store Write1/7
  BinarySwitch14/1 -> HardwareInputControl14/1
  HardwareInputControl14/1 -> Data Store Write5/7
  BinarySwitch25/1 -> HardwareInputControl25/1
  HardwareInputControl25/1 -> Data Store Write5/1
  HardwareInputControl26/1 -> Data Store Write1/12
  BinarySwitch26/1 -> HardwareInputControl26/1
  BinarySwitch27/1 -> HardwareInputControl27/1
  HardwareInputControl27/1 -> Data Store Write1/1
  HardwareInputControl15/1 -> Data Store Write2/1
  BinarySwitch15/1 -> HardwareInputControl15/1
  BinarySwitch13/1 -> HardwareInputControl13/1
  HardwareInputControl13/1 -> Data Store Write2/24, Data Store Write2/23, Data Store Write2/22, Data Store Write2/21, Data Store Write2/20, Data Store Write2/19, Data Store Write2/18, Data Store Write2/17, Data Store Write2/16, Data Store Write2/15, Data Store Write2/14, Data Store Write2/13, Data Store Write2/12
  HardwareInputControl9/1 -> Data Store Write2/7
  BinarySwitch9/1 -> HardwareInputControl9/1
  HardwareInputControl2/1 -> Data Store Write2/11, Data Store Write2/10, Data Store Write2/9, Data Store Write2/8, Data Store Write2/6, Data Store Write2/5, Data Store Write2/4, Data Store Write2/3, Data Store Write2/2
  BinarySwitch2/1 -> HardwareInputControl2/1
  HardwareInputControl16/1 -> Data Store Write6/12
  BinarySwitch16/1 -> HardwareInputControl16/1
  HardwareInputControl18/1 -> Data Store Write7/1
  BinarySwitch18/1 -> HardwareInputControl18/1
  BinarySwitch19/1 -> HardwareInputControl19/1
  HardwareInputControl19/1 -> Data Store Write7/2
  HardwareInputControl20/1 -> Data Store Write7/4
  BinarySwitch20/1 -> HardwareInputControl20/1
  BinarySwitch17/1 -> HardwareInputControl17/1
  HardwareInputControl17/1 -> Data Store Write7/3

== system BEML_EMU_TestBench_6Car/Subsystem/LightingTest ==
  In1 : Inport
  Bus Selector : BusSelector  OutputSignals=OutputControlStates.HeadLight,OutputControlStates.MarkerOrTailLight,OutputControlStates.FloodLight,OutputControlStates.FlasherLight,OutputControlStates.UTOOrRMLight
  Bus Selector1 : BusSelector  Commented=on  OutputSignals=OutputControlStates.DirIndicatorLeft,OutputControlStates.DirIndicatorRight
  Bus Selector2 : BusSelector  Commented=on  OutputSignals=OutputControlStates.DirIndicatorLeft,OutputControlStates.DirIndicatorRight
  Bus Selector3 : BusSelector  OutputSignals=OutputControlStates.HeadLight,OutputControlStates.MarkerOrTailLight,OutputControlStates.FloodLight,OutputControlStates.FlasherLight,OutputControlStates.UTOOrRMLight
  DMC1 : Selector  InputPortWidth=MaxVehicles  IndexOptions=Index vector (dialog)  Indices=1  OutputSizes=1
  DMC2 : Selector  InputPortWidth=MaxVehicles  IndexOptions=Index vector (dialog)  Indices=6  OutputSizes=1
  Display1 : Display
  Display{2..5} (4 alike) : Display  Commented=on
  Display6 : Display
  M1 : Selector  Commented=on  InputPortWidth=MaxVehicles  IndexOptions=Index vector (dialog)  Indices=3  OutputSizes=1
  T1 : Selector  Commented=on  InputPortWidth=MaxVehicles  IndexOptions=Index vector (dialog)  Indices=2  OutputSizes=1
  Vector Concatenate : Concatenate  NumInputs=5
  Vector Concatenate1 : Concatenate  NumInputs=5
  wires:
  In1/1 -> DMC2/1, M1/1, T1/1, DMC1/1
  DMC1/1 -> Bus Selector/1
  Bus Selector/1 -> Vector Concatenate/1  "<HeadLight>"
  Bus Selector/2 -> Vector Concatenate/2  "<MarkerOrTailLight>"
  Bus Selector1/2 -> Display3/1  "<DirIndicatorRight>"
  Bus Selector1/1 -> Display2/1  "<DirIndicatorLeft>"
  T1/1 -> Bus Selector1/1
  DMC2/1 -> Bus Selector3/1
  Bus Selector2/2 -> Display5/1  "<DirIndicatorRight>"
  Bus Selector2/1 -> Display4/1  "<DirIndicatorLeft>"
  M1/1 -> Bus Selector2/1
  Bus Selector/4 -> Vector Concatenate/4  "<FlasherLight>"
  Bus Selector/5 -> Vector Concatenate/5  "<UTOOrRMLight>"
  Bus Selector/3 -> Vector Concatenate/3  "<FloodLight>"
  Vector Concatenate/1 -> Display1/1
  Bus Selector3/1 -> Vector Concatenate1/1  "<HeadLight>"
  Vector Concatenate1/1 -> Display6/1
  Bus Selector3/5 -> Vector Concatenate1/5  "<UTOOrRMLight>"
  Bus Selector3/3 -> Vector Concatenate1/3  "<FloodLight>"
  Bus Selector3/4 -> Vector Concatenate1/4  "<FlasherLight>"
  Bus Selector3/2 -> Vector Concatenate1/2  "<MarkerOrTailLight>"

== system BEML_EMU_TestBench_6Car/Subsystem/MotionBaseController ==
  MotionBaseOut : Inport
  BinarySwitch26 : TestBenchLib/BinarySwitch  value=0  init_value=0  block_colour=[0 1 0]  WorkspaceVarName=0
      settings: SourceProductName=Sydac Utilities
  Bus Selector2 : BusSelector  OutputSignals=LinearVelocity,LinearAcceleration,AngularVelocity,AngularAcceleration
  DMC2 : Selector  InputPortWidth=MaxVehicles  IndexOptions=Index vector (dialog)  Indices=6  OutputSizes=1
  Data Store Write5 : DataStoreWrite  DataStoreName=MotionBaseControllerInput  DataStoreElements=MotionBaseControllerInput(6).Effects.OnRoughTrack
  Scope : Scope  NumInputPorts=4
  wires:
  BinarySwitch26/1 -> Data Store Write5/1
  DMC2/1 -> Bus Selector2/1
  MotionBaseOut/1 -> DMC2/1
  Bus Selector2/1 -> Scope/1  "<LinearVelocity>"
  Bus Selector2/2 -> Scope/2  "<LinearAcceleration>"
  Bus Selector2/3 -> Scope/3  "<AngularVelocity>"
  Bus Selector2/4 -> Scope/4  "<AngularAcceleration>"

== system BEML_EMU_TestBench_6Car/Subsystem/PneumaticSystemDashboard ==
  In1 : Inport
  Bus Selector1 : BusSelector  OutputSignals=Bogie
  Bus Selector10 : BusSelector  OutputSignals=PressureGauges
  Bus Selector14 : BusSelector  OutputSignals=MainReservoirPressureGauge,SRPressureGauge
  Bus Selector17 : BusSelector  OutputSignals=BrakeReservoirPressureSwitch,PS3,MainReservoirPipePressureSwitch,MainReservoirPressureSwitch
  Bus Selector19 : BusSelector  OutputSignals=PressureSwitches
  Bus Selector3 : BusSelector  OutputSignals=PressureSwitches.VCBPressureSwitch,PressureGauges.MainReservoirPressureGauge,PressureGauges.SRPressureGauge
  Bus Selector4 : BusSelector  OutputSignals=BrakeCylinderPressureGauge,ParkBrakePressureGauge
  Bus Selector5 : BusSelector  OutputSignals=Bogie
  Bus Selector6 : BusSelector  OutputSignals=ParkBrakePressureSwitch
  DMC2 : Selector  InputPortWidth=MaxVehicles  IndexOptions=Index vector (dialog)  Indices=6  OutputSizes=1
  DMC2. : Selector  InputPortWidth=MaxVehicles  IndexOptions=Index vector (dialog)  Indices=6  OutputSizes=1
  Data Type Conversion3 : DataTypeConversion  Commented=through
  Display{1..2,4..6,15,19} (7 alike) : Display
  Mux1 : Mux  Inputs=3
  Mux3 : Mux
  Scope1 : Scope  Commented=on
  Tc1 : Selector  InputPortWidth=MaxVehicles  IndexOptions=Index vector (dialog)  Indices=2  OutputSizes=1
  Tc3 : Selector  NumberOfDimensions=2  InputPortWidth=MaxVehicles  IndexOptions=Index vector (dialog),Index vector (dialog)  Indices=1,2  OutputSizes=1,1
  Tc4 : Selector  NumberOfDimensions=2  InputPortWidth=MaxVehicles  IndexOptions=Index vector (dialog),Index vector (dialog)  Indices=1,2  OutputSizes=1,1
  wires:
  Data Type Conversion3/1 -> Mux3/1
  Bus Selector4/1 -> Scope1/1, Display1/1  "<BrakeCylinderPressureGauge>"
  Bus Selector14/2 -> Display2/1  "<SRPressureGauge>"
  Bus Selector5/1 -> Tc4/1  "<Bogie>"
  Bus Selector19/1 -> Bus Selector5/1, Bus Selector17/1  "<PressureSwitches>"
  DMC2./1 -> Bus Selector19/1
  Bus Selector6/1 -> Display5/1  "<ParkBrakePressureSwitch>"
  Tc4/1 -> Bus Selector6/1
  Tc3/1 -> Bus Selector4/1
  Bus Selector17/1 -> Data Type Conversion3/1  "<BrakeReservoirPressureSwitch>"
  Bus Selector3/2 -> Mux1/2  "<MainReservoirPressureGauge>"
  Bus Selector17/3 -> Mux3/3  "<MainReservoirPipePressureSwitch>"
  Bus Selector14/1 -> Display19/1  "<MainReservoirPressureGauge>"
  In1/1 -> Tc1/1, DMC2/1, DMC2./1
  Bus Selector4/2 -> Display4/1  "<ParkBrakePressureGauge>"
  Bus Selector17/4 -> Mux3/4  "<MainReservoirPressureSwitch>"
  Tc1/1 -> Bus Selector3/1
  Bus Selector3/1 -> Mux1/1  "<VCBPressureSwitch>"
  DMC2/1 -> Bus Selector10/1
  Mux1/1 -> Display6/1
  Bus Selector3/3 -> Mux1/3  "<SRPressureGauge>"
  Bus Selector10/1 -> Bus Selector14/1, Bus Selector1/1  "<PressureGauges>"
  Bus Selector1/1 -> Tc3/1  "<Bogie>"
  Mux3/1 -> Display15/1
  Bus Selector17/2 -> Mux3/2  "<PS3>"

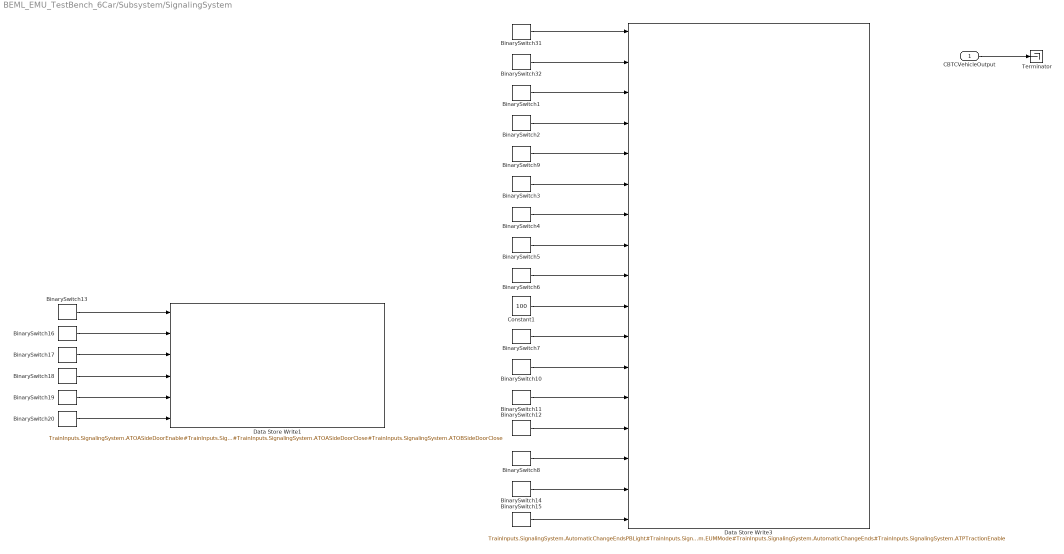
== system BEML_EMU_TestBench_6Car/Subsystem/SignalingSystem ==
  CBTCVehicleOutput : Inport
  BinarySwitch{1..20,31..32} (22 alike) : TestBenchLib/BinarySwitch  value=0  init_value=0  block_colour=[0 1 0]  WorkspaceVarName=0
      settings: SourceProductName=Sydac Utilities
  Constant1 : Constant  Value=100
  Data Store Write1 : DataStoreWrite  Priority=1  DataStoreName=TrainInputs  DataStoreElements=TrainInputs.SignalingSystem.ATOASideDoorEnable#TrainInputs.SignalingSystem.ATOBSideDoorEnable#TrainInputs.SignalingSystem.ATOASideDoorOpen#TrainInputs.SignalingSystem.ATOBSideDoorOpen#TrainInputs.SignalingSystem.ATOASideDoorClose#TrainInputs.SignalingSystem.ATOBSideDoorClose
  Data Store Write3 : DataStoreWrite  Priority=1  DataStoreName=TrainInputs  DataStoreElements=TrainInputs.SignalingSystem.AutomaticChangeEndsPBLight#TrainInputs.SignalingSystem.ATOStartPBLight#TrainInputs.SignalingSystem.ATOActivate#TrainInputs.SignalingSystem.ATOForward#TrainInputs.SignalingSystem.ATCZeroSpeed#TrainInputs.SignalingSystem.ATOTraction#TrainInputs.SignalingSystem.ATPEmergencyBrake#TrainInputs.SignalingSystem.ATOHoldingBrake#TrainInputs.SignalingSystem.ATOBrake#TrainInputs.SignalingSystem.ATOTractionBrakeDemand#TrainInputs.SignalingSystem.ATORear#TrainInputs.SignalingSystem.RMMode#TrainInputs.SignalingSystem.CMMode#TrainInputs.SignalingSystem.AMMode#TrainInputs.SignalingSystem.EUMMode#TrainInputs.SignalingSystem.AutomaticChangeEnds#TrainInputs.SignalingSystem.ATPTractionEnable
  Terminator : Terminator
  wires:
  CBTCVehicleOutput/1 -> Terminator/1
  BinarySwitch31/1 -> Data Store Write3/1
  BinarySwitch32/1 -> Data Store Write3/2
  BinarySwitch1/1 -> Data Store Write3/3
  BinarySwitch2/1 -> Data Store Write3/4
  Constant1/1 -> Data Store Write3/10
  BinarySwitch6/1 -> Data Store Write3/9
  BinarySwitch5/1 -> Data Store Write3/8
  BinarySwitch4/1 -> Data Store Write3/7
  BinarySwitch3/1 -> Data Store Write3/6
  BinarySwitch9/1 -> Data Store Write3/5
  BinarySwitch10/1 -> Data Store Write3/12
  BinarySwitch11/1 -> Data Store Write3/13
  BinarySwitch12/1 -> Data Store Write3/14
  BinarySwitch8/1 -> Data Store Write3/15
  BinarySwitch14/1 -> Data Store Write3/16
  BinarySwitch15/1 -> Data Store Write3/17
  BinarySwitch13/1 -> Data Store Write1/1
  BinarySwitch16/1 -> Data Store Write1/2
  BinarySwitch17/1 -> Data Store Write1/3
  BinarySwitch18/1 -> Data Store Write1/4
  BinarySwitch19/1 -> Data Store Write1/5
  BinarySwitch20/1 -> Data Store Write1/6
  BinarySwitch7/1 -> Data Store Write3/11

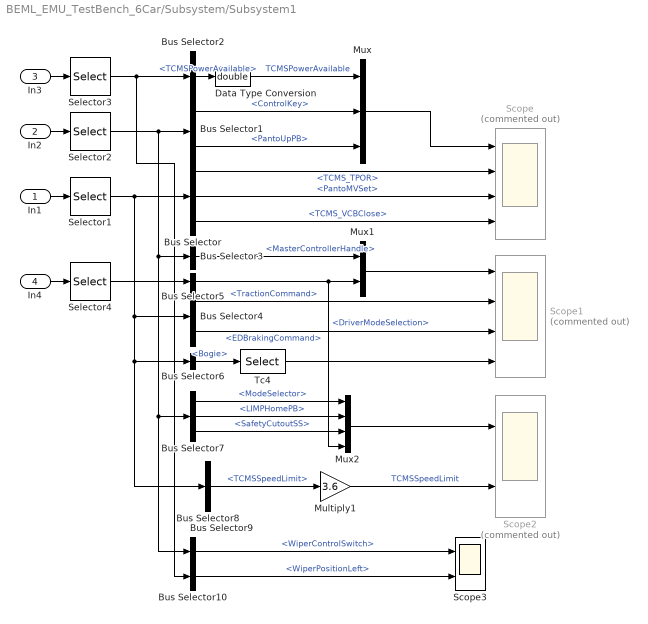
== system BEML_EMU_TestBench_6Car/Subsystem/Subsystem1 ==
  In1 : Inport
  In2 : Inport  Port=2
  In3 : Inport  Port=3
  In4 : Inport  Port=4
  Bus Selector : BusSelector  OutputSignals=Control.ElectricalSystem.TCMS_TPOR,Control.ElectricalSystem.PantoMVSet,Control.ElectricalSystem.TCMS_VCBClose
  Bus Selector1 : BusSelector  OutputSignals=InputStates.ControlKey,InputStates.PantoUpPB
  Bus Selector10 : BusSelector  OutputSignals=OutputControlStates.WiperPositionLeft
  Bus Selector2 : BusSelector  OutputSignals=TCMS.TCMSPowerAvailable
  Bus Selector3 : BusSelector  OutputSignals=InputStates.MasterControllerHandle
  Bus Selector4 : BusSelector  OutputSignals=Control.TractionSBraking.TractionCommand,Control.TractionSBraking.EDBrakingCommand
  Bus Selector5 : BusSelector  OutputSignals=OnBoard.DriverModeSelection
  Bus Selector6 : BusSelector  OutputSignals=Control.TractionSBraking.Bogie
  Bus Selector7 : BusSelector  OutputSignals=InputStates.ModeSelector,InputStates.LIMPHomePB,InputStates.SafetyCutoutSS
  Bus Selector8 : BusSelector  OutputSignals=Display.TractionBraking.TCMSSpeedLimit
  Bus Selector9 : BusSelector  OutputSignals=InputStates.WiperControlSwitch
  Data Type Conversion : DataTypeConversion  OutDataTypeStr=double
  Multiply1 : Gain  Gain=3.6
  Mux : Mux  Inputs=3
  Mux1 : Mux  Inputs=2
  Mux2 : Mux
  Scope : Scope  Commented=on  NumInputPorts=4
  Scope1 : Scope  Commented=on  NumInputPorts=4
  Scope2 : Scope  Commented=on  NumInputPorts=2
  Scope3 : Scope  NumInputPorts=2
  Selector{1..4} (4 alike) : Selector  InputPortWidth=MaxVehicles  IndexOptions=Index vector (dialog)  Indices=6  OutputSizes=1
  Tc4 : Selector  NumberOfDimensions=2  InputPortWidth=MaxVehicles  IndexOptions=Index vector (dialog),Index vector (dialog)  Indices=1,1  OutputSizes=1,1
  wires:
  Selector1/1 -> Bus Selector8/1, Bus Selector6/1, Bus Selector4/1, Bus Selector/1
  In1/1 -> Selector1/1
  Bus Selector/1 -> Scope/2  "<TCMS_TPOR>"
  Bus Selector/2 -> Scope/3  "<PantoMVSet>"
  Bus Selector/3 -> Scope/4  "<TCMS_VCBClose>"
  In2/1 -> Selector2/1
  Selector2/1 -> Bus Selector9/1, Bus Selector7/1, Bus Selector3/1, Bus Selector1/1
  Bus Selector1/1 -> Mux/2  "<ControlKey>"
  Bus Selector1/2 -> Mux/3  "<PantoUpPB>"
  Mux/1 -> Scope/1
  In3/1 -> Selector3/1
  Selector3/1 -> Bus Selector10/1, Bus Selector2/1
  Bus Selector2/1 -> Data Type Conversion/1  "<TCMSPowerAvailable>"
  Data Type Conversion/1 -> Mux/1  "TCMSPowerAvailable"
  Bus Selector3/1 -> Mux1/1  "<MasterControllerHandle>"
  Bus Selector4/1 -> Scope1/2  "<TractionCommand>"
  Bus Selector4/2 -> Scope1/3  "<EDBrakingCommand>"
  Tc4/1 -> Scope1/4
  In4/1 -> Selector4/1
  Selector4/1 -> Bus Selector5/1
  Bus Selector5/1 -> Mux2/4, Mux1/2  "<DriverModeSelection>"
  Mux1/1 -> Scope1/1
  Bus Selector6/1 -> Tc4/1  "<Bogie>"
  Mux2/1 -> Scope2/1
  Bus Selector7/1 -> Mux2/1  "<ModeSelector>"
  Bus Selector7/2 -> Mux2/2  "<LIMPHomePB>"
  Bus Selector7/3 -> Mux2/3  "<SafetyCutoutSS>"
  Bus Selector8/1 -> Multiply1/1  "<TCMSSpeedLimit>"
  Multiply1/1 -> Scope2/2  "TCMSSpeedLimit"
  Bus Selector9/1 -> Scope3/1  "<WiperControlSwitch>"
  Bus Selector10/1 -> Scope3/2  "<WiperPositionLeft>"
